simulink library "RGP_objF_ul"  (R2018b)
settings: Solver=VariableStepAuto  StartTime=0.0  StopTime=10.0  RelTol=1e-3
undefined symbols (not defined in the file or in its folder): turbRatedSpeed
libraries: simulink x2, dspsigops x2
settings Model: Creator=Ayaz  LastModifiedBy=Ayaz
settings DataIOCC: ReturnWorkspaceOutputs=on

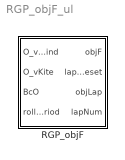
== system RGP_objF_ul ==
  RGP_objF : Subsystem  mask{vRated=turbRatedSpeed}
      mask prompts: vRated "Turbine rated speed [m/s]"
      mask TypeOptions vRated: Constant4/Value

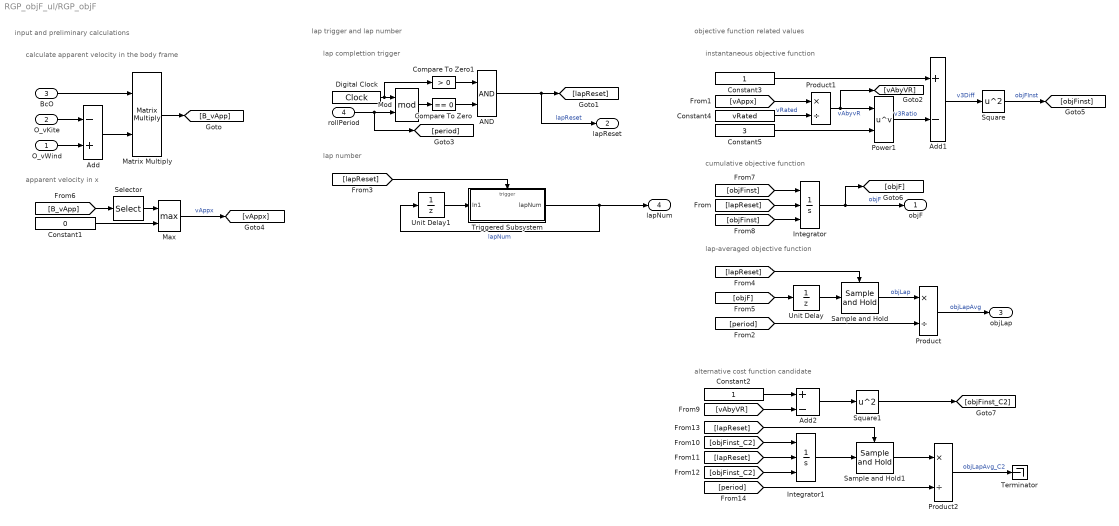
== system RGP_objF_ul/RGP_objF ==
  note: alternative cost function candidate
  note: input and preliminary calculations
  note: objective function related values
  note: lap-averaged objective function
  note: lap trigger and lap number
  note: lap complettion trigger
  note: apparent velocity in x
  note: cumulative objective function
  note: instantaneous objective function
  note: lap number
  note: calculate apparent velocity in the body frame
  O_vWind : Inport
  O_vKite : Inport  Port=2
  BcO : Inport  Port=3
  rollPeriod : Inport  Port=4
  AND : Logic  AllPortsSameDT=off  OutDataTypeStr=boolean
  Add : Sum  Inputs=-+
  Add1 : Sum  Inputs=+-
  Add2 : Sum  Inputs=+-
  Compare To Zero : simulink/Logic and Bit Operations/Compare To Zero  relop===  OutDataTypeStr=boolean
  Compare To Zero1 : simulink/Logic and Bit Operations/Compare To Zero  relop=>  OutDataTypeStr=boolean
  Constant1 : Constant  Value=0  VectorParams1D=off
  Constant2 : Constant
  Constant3 : Constant
  Constant4 : Constant  Value=vRated  VectorParams1D=off
  Constant5 : Constant  Value=3
  Digital Clock : DigitalClock
  Integrator : Integrator  ExternalReset=rising  InitialConditionSource=external
  Integrator1 : Integrator  ExternalReset=rising  InitialConditionSource=external
  Matrix Multiply : Product  Multiplication=Matrix(*)
  Max : MinMax  Function=max  Inputs=2
  Mod : Math  Operator=mod  SaturateOnIntegerOverflow=on
  Power1 : Math  Operator=pow  SaturateOnIntegerOverflow=on
  Product : Product  Inputs=*/
  Product1 : Product  Inputs=*/
  Product2 : Product  Inputs=*/
  Sample and Hold : dspsigops/Sample and Hold  trig=Rising edge  initCond=0  latchinput=off
  Sample and Hold1 : dspsigops/Sample and Hold  trig=Rising edge  initCond=0  latchinput=off
  Selector : Selector  InputPortWidth=3  IndexOptions=Index vector (dialog)  Indices=1  OutputSizes=1
  Square : Math  Operator=square  SaturateOnIntegerOverflow=on
  Square1 : Math  Operator=square  SaturateOnIntegerOverflow=on
  Terminator : Terminator
  Triggered Subsystem : Subsystem  TreatAsAtomicUnit=on
  Unit Delay : UnitDelay  SampleTime=-1  HasFrameUpgradeWarning=on
  Unit Delay1 : UnitDelay  SampleTime=-1  HasFrameUpgradeWarning=on
  objF : Outport
  lapReset : Outport  Port=2
  objLap : Outport  Port=3
  lapNum : Outport  Port=4
  wires:
  O_vKite/1 -> Add/1
  O_vWind/1 -> Add/2
  Add/1 -> Matrix Multiply/2
  BcO/1 -> Matrix Multiply/1
  Max/1 -> [vAppx]  "vAppx"
  Constant1/1 -> Max/2
  Matrix Multiply/1 -> [B_vApp]
  Selector/1 -> Max/1
  [B_vApp] -> Selector/1
  [lapReset] -> Integrator/2
  [vAppx] -> Product1/1
  Integrator/1 -> objF/1, [objF]  "objF"
  Add1/1 -> Square/1  "v3Diff"
  [lapReset] -> Sample and Hold/Trigger
  Sample and Hold/1 -> Product/1  "objLap"
  [objF] -> Unit Delay/1
  AND/1 -> lapReset/1, [lapReset]  "lapReset"
  Unit Delay/1 -> Sample and Hold/1
  Product/1 -> objLap/1  "objLapAvg"
  Power1/1 -> Add1/2  "v3Ratio"
  Constant3/1 -> Add1/1
  Digital Clock/1 -> Compare To Zero1/1, Mod/1
  rollPeriod/1 -> [period], Mod/2
  Mod/1 -> Compare To Zero/1
  [period] -> Product/2
  Compare To Zero1/1 -> AND/1
  Compare To Zero/1 -> AND/2
  [lapReset] -> Triggered Subsystem/Trigger
  Unit Delay1/1 -> Triggered Subsystem/1(In1)
  Triggered Subsystem/1(lapNum) -> lapNum/1, Unit Delay1/1  "lapNum"
  Product1/1 -> [vAbyVR], Power1/1  "vAbyvR"
  Constant5/1 -> Power1/2
  Square/1 -> [objFinst]  "objFInst"
  [objFinst] -> Integrator/1
  [objFinst] -> Integrator/3
  Constant4/1 -> Product1/2  "vRated"
  Constant2/1 -> Add2/1
  [vAbyVR] -> Add2/2
  Add2/1 -> Square1/1
  Square1/1 -> [objFinst_C2]
  [objFinst_C2] -> Integrator1/1
  [lapReset] -> Integrator1/2
  [objFinst_C2] -> Integrator1/3
  Integrator1/1 -> Sample and Hold1/1
  [lapReset] -> Sample and Hold1/Trigger
  Sample and Hold1/1 -> Product2/1
  [period] -> Product2/2
  Product2/1 -> Terminator/1  "objLapAvg_C2"

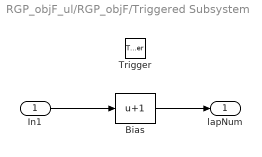
== system RGP_objF_ul/RGP_objF/Triggered Subsystem ==
  In1 : Inport
  Trigger : TriggerPort  VariantControl=Variant
  Bias : Bias  Bias=1
  lapNum : Outport
  wires:
  In1/1 -> Bias/1
  Bias/1 -> lapNum/1
